simulink model "model_dyskretny_2_reg_obs"  (R2020a)
settings: Solver=VariableStepAuto  StartTime=0.0  StopTime=10.0  RelTol=1e-3
values from neighbouring files (symbols this model uses):
  K = acker(A,B, [zb1, zb2, zb3])    [zad1_10.m]    (also in zad1_6.m = [k1 k2 k3]; zad1_6_1.m = acker(A,B, [zb(3), zb(3), zb(3)]); zad1_6_2.m = acker(A,B, [zb1, complex(a(1), b(3)), complex(a(1), -b(3))]); zad1_9.m)
  L = acker(A22',A12', [zo(2), zo(2)])'    [zad1_10.m]    (also in zad1_9.m)
  T = 0.5    [pom.m]    (also in zad1_10.m; zad1_4.m; zad1_6_1.m; zad1_6_2.m)
  u2z = B2-L*B1    [zad1_10.m]    (also in zad1_9.m)
  y2z = (A22-L*A12)*L + A21-L*A11    [zad1_10.m]    (also in zad1_9.m)
  z2z = A22-L*A12    [zad1_10.m]    (also in zad1_9.m)
settings Model: Creator=jakub  LastModifiedBy=jakub
settings DebuggingCC: InitInArrayFormatMsg=none

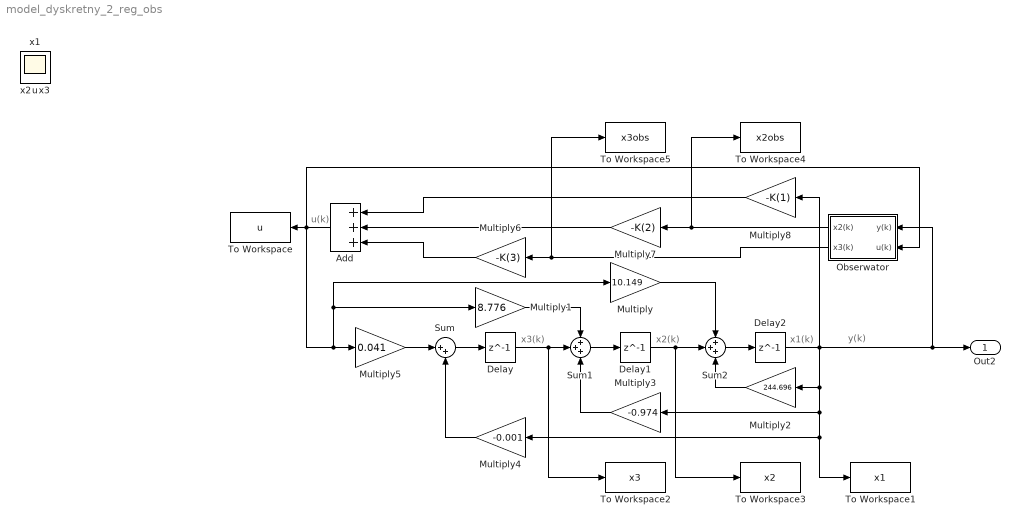
== system model_dyskretny_2_reg_obs ==
  note: y(k)
  note: u(k)
  note: x2(k)
  note: x3(k)
  note: x1(k)
  Add : Sum  Inputs=+++
  Delay : Delay  DelayLength=1  InitialCondition=5  SampleTime=T
  Delay1 : Delay  DelayLength=1  InitialCondition=-2  SampleTime=T
  Delay2 : Delay  DelayLength=1  InitialCondition=-1  SampleTime=T
  Multiply : Gain  Gain=10.149
  Multiply1 : Gain  Gain=8.776
  Multiply2 : Gain  Gain=244.696
  Multiply3 : Gain  Gain=-0.974
  Multiply4 : Gain  Gain=-0.001
  Multiply5 : Gain  Gain=0.041
  Multiply6 : Gain  Gain=-K(3)
  Multiply7 : Gain  Gain=-K(2)
  Multiply8 : Gain  Gain=-K(1)
  Obserwator : Subsystem
  Sum : Sum  Inputs=|++
  Sum1 : Sum  Inputs=+++
  Sum2 : Sum  Inputs=+++
  To Workspace : ToWorkspace  VariableName=u  SaveFormat=Structure With Time  SampleTime=-1
  To Workspace1 : ToWorkspace  VariableName=x1  SaveFormat=Structure With Time  SampleTime=-1
  To Workspace2 : ToWorkspace  VariableName=x3  SaveFormat=Structure With Time  SampleTime=-1
  To Workspace3 : ToWorkspace  VariableName=x2  SaveFormat=Structure With Time  SampleTime=-1
  To Workspace4 : ToWorkspace  VariableName=x2obs  SaveFormat=Structure With Time  SampleTime=-1
  To Workspace5 : ToWorkspace  VariableName=x3obs  SaveFormat=Structure With Time  SampleTime=-1
  Out2 : Outport
  u : Scope
  x1 : Scope
  x2 : Scope
  x3 : Scope
  wires:
  Add/1 -> Obserwator/2(u(k)), To Workspace/1, Multiply/1, Multiply1/1, Multiply5/1
  Sum/1 -> Delay/1
  Multiply5/1 -> Sum/1
  Sum1/1 -> Delay1/1
  Delay1/1 -> To Workspace3/1, Sum2/2
  Sum2/1 -> Delay2/1
  Delay/1 -> To Workspace2/1, Sum1/2
  Delay2/1 -> To Workspace1/1, Multiply4/1, Multiply3/1, Multiply2/1, Multiply8/1, Obserwator/1(y(k)), Out2/1
  Multiply1/1 -> Sum1/1
  Multiply/1 -> Sum2/1
  Multiply3/1 -> Sum1/3
  Multiply4/1 -> Sum/2
  Multiply2/1 -> Sum2/3
  Multiply8/1 -> Add/1
  Multiply7/1 -> Add/2
  Multiply6/1 -> Add/3
  Obserwator/1(x2(k)) -> To Workspace4/1, Multiply7/1
  Obserwator/2(x3(k)) -> To Workspace5/1, Multiply6/1

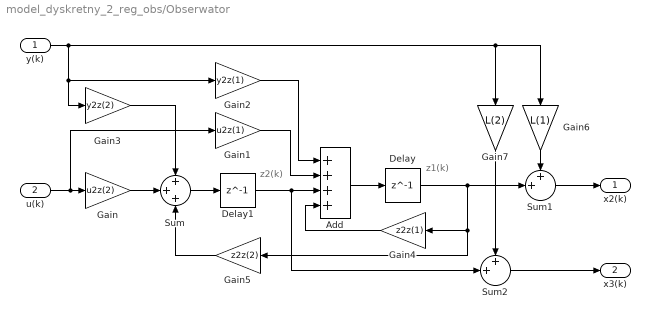
== system model_dyskretny_2_reg_obs/Obserwator ==
  note: z2(k)
  note: z1(k)
  y(k) : Inport
  u(k) : Inport  Port=2
  Add : Sum  Inputs=++++
  Delay : Delay  DelayLength=1  InitialCondition=0
  Delay1 : Delay  DelayLength=1  InitialCondition=0
  Gain : Gain  Gain=u2z(2)
  Gain1 : Gain  Gain=u2z(1)
  Gain2 : Gain  Gain=y2z(1)
  Gain3 : Gain  Gain=y2z(2)
  Gain4 : Gain  Gain=z2z(1)
  Gain5 : Gain  Gain=z2z(2)
  Gain6 : Gain  Gain=L(1)
  Gain7 : Gain  Gain=L(2)
  Sum : Sum  Inputs=+++
  Sum1 : Sum  Inputs=++|
  Sum2 : Sum  Inputs=++|
  x2(k) : Outport
  x3(k) : Outport  Port=2
  wires:
  Gain7/1 -> Sum2/1
  Gain6/1 -> Sum1/1
  Gain4/1 -> Add/4
  Sum1/1 -> x2(k)/1
  Sum2/1 -> x3(k)/1
  Gain2/1 -> Add/1
  u(k)/1 -> Gain1/1, Gain/1
  Gain5/1 -> Sum/3
  y(k)/1 -> Gain2/1, Gain3/1, Gain7/1, Gain6/1
  Sum/1 -> Delay1/1
  Gain/1 -> Sum/2
  Gain1/1 -> Add/2
  Gain3/1 -> Sum/1
  Add/1 -> Delay/1
  Delay/1 -> Sum1/2, Gain5/1, Gain4/1
  Delay1/1 -> Sum2/2, Add/3
